simulink model "V2G_Simulator"  (R2021b)
settings: Solver=VariableStepAuto  StartTime=0.0  StopTime=10.0  RelTol=1e-3
settings Model: Creator=The MathWorks, Inc.  LastModifiedBy=rhdej

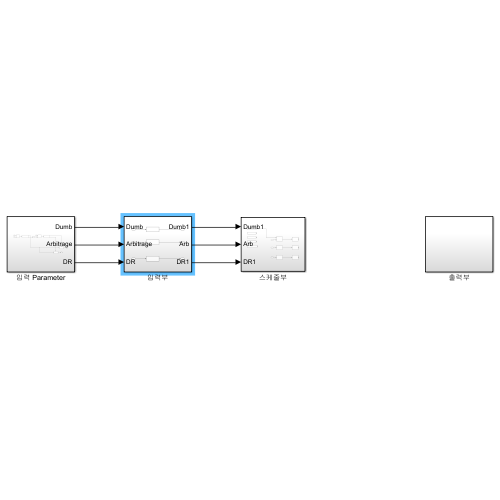
[thumbnail: Simulink's stored preview of the top-level diagram]
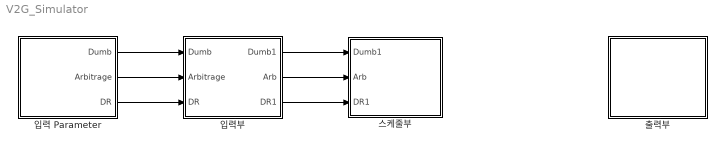
== system V2G_Simulator ==
  스케줄부 : Subsystem
  입력 Parameter : Subsystem
  입력부 : Subsystem
  출력부 : Subsystem
  wires:
  입력부/1(Dumb1) -> 스케줄부/1(Dumb1)
  입력부/2(Arb) -> 스케줄부/2(Arb)
  입력부/3(DR1) -> 스케줄부/3(DR1)
  입력 Parameter/1(Dumb) -> 입력부/1(Dumb)
  입력 Parameter/2(Arbitrage) -> 입력부/2(Arbitrage)
  입력 Parameter/3(DR) -> 입력부/3(DR)

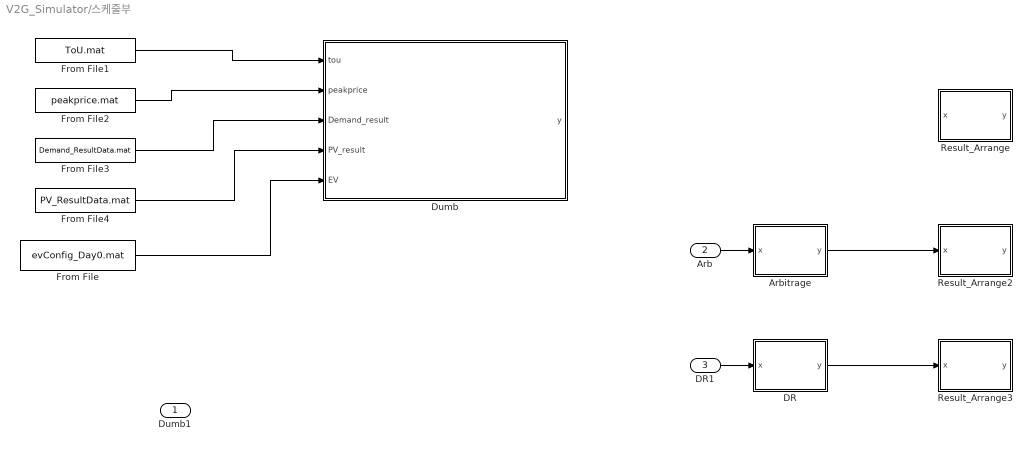
== system V2G_Simulator/스케줄부 ==
  Dumb1 : Inport
  Arb : Inport  Port=2
  DR1 : Inport  Port=3
  Arbitrage : MATLAB Function  TreatAsAtomicUnit=on
  DR : MATLAB Function  TreatAsAtomicUnit=on
  Dumb : MATLAB Function  TreatAsAtomicUnit=on
  From File : FromFile  FileName=evConfig_Day0.mat  SampleTime=0
  From File1 : FromFile  FileName=ToU.mat  SampleTime=0
  From File2 : FromFile  FileName=peakprice.mat  SampleTime=0
  From File3 : FromFile  FileName=Demand_ResultData.mat  SampleTime=0
  From File4 : FromFile  FileName=PV_ResultData.mat  SampleTime=0
  Result_Arrange : MATLAB Function  TreatAsAtomicUnit=on
  Result_Arrange2 : MATLAB Function  TreatAsAtomicUnit=on
  Result_Arrange3 : MATLAB Function  TreatAsAtomicUnit=on
  wires:
  Arbitrage/1(y) -> Result_Arrange2/1(x)
  DR/1(y) -> Result_Arrange3/1(x)
  Arb/1 -> Arbitrage/1(x)
  DR1/1 -> DR/1(x)
  From File1/1 -> Dumb/1(tou)
  From File2/1 -> Dumb/2(peakprice)
  From File3/1 -> Dumb/3(Demand_result)
  From File4/1 -> Dumb/4(PV_result)
  From File/1 -> Dumb/5(EV)

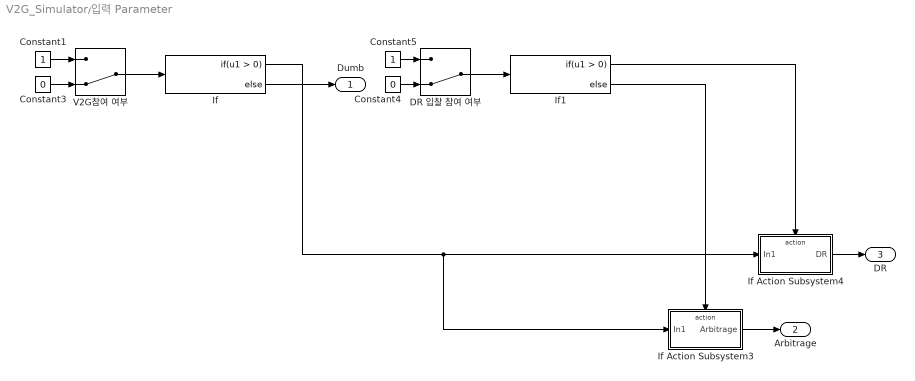
== system V2G_Simulator/입력 Parameter ==
  Constant1 : Constant
  Constant3 : Constant  Value=0
  Constant4 : Constant  Value=0
  Constant5 : Constant
  DR 입찰 참여 여부 : ManualSwitch  CurrentSetting=0
  If : If
  If Action Subsystem3 : Subsystem  TreatAsAtomicUnit=on
  If Action Subsystem4 : Subsystem  TreatAsAtomicUnit=on
  If1 : If
  V2G참여 여부 : ManualSwitch  CurrentSetting=0
  Dumb : Outport
  Arbitrage : Outport  Port=2
  DR : Outport  Port=3
  wires:
  Constant3/1 -> V2G참여 여부/2
  Constant1/1 -> V2G참여 여부/1
  V2G참여 여부/1 -> If/1
  If/2 -> Dumb/1
  Constant4/1 -> DR 입찰 참여 여부/2
  Constant5/1 -> DR 입찰 참여 여부/1
  DR 입찰 참여 여부/1 -> If1/1
  If/1 -> If Action Subsystem4/1(In1), If Action Subsystem3/1(In1)
  If1/2 -> If Action Subsystem3/Action
  If Action Subsystem4/1(DR) -> DR/1
  If Action Subsystem3/1(Arbitrage) -> Arbitrage/1
  If1/1 -> If Action Subsystem4/Action

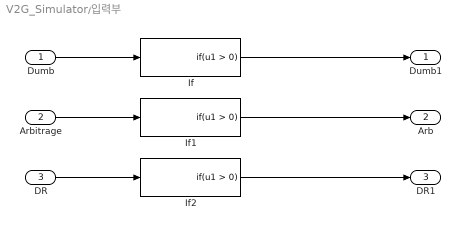
== system V2G_Simulator/입력부 ==
  Dumb : Inport
  Arbitrage : Inport  Port=2
  DR : Inport  Port=3
  If : If  ShowElse=off
  If1 : If  ShowElse=off
  If2 : If  ShowElse=off
  Dumb1 : Outport
  Arb : Outport  Port=2
  DR1 : Outport  Port=3
  wires:
  Dumb/1 -> If/1
  Arbitrage/1 -> If1/1
  DR/1 -> If2/1
  If/1 -> Dumb1/1
  If1/1 -> Arb/1
  If2/1 -> DR1/1

== system V2G_Simulator/출력부 ==

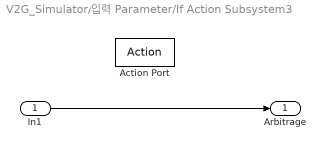
== system V2G_Simulator/입력 Parameter/If Action Subsystem3 ==
  In1 : Inport
  Action Port : ActionPort  ActionPortLabel=else
  Arbitrage : Outport
  wires:
  In1/1 -> Arbitrage/1

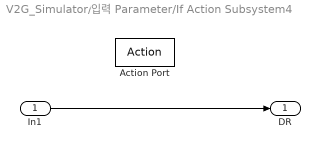
== system V2G_Simulator/입력 Parameter/If Action Subsystem4 ==
  In1 : Inport
  Action Port : ActionPort  ActionPortLabel=if(u1 > 0)
  DR : Outport
  wires:
  In1/1 -> DR/1

== matlab function V2G_Simulator/스케줄부/Arbitrage ==
  data: x input; y output
function y = temp(x)


end

== matlab function V2G_Simulator/스케줄부/DR ==
  data: x input; y output
function y = temp(x)

== matlab function V2G_Simulator/스케줄부/Dumb ==
  data: tou input; y output; peakprice input; Demand_result input; PV_result input; EV input
function y = temp(tou, peakprice, Demand_result, PV_result, EV)

coder.extrinsic("intlinprog")

x = [0]


end

== matlab function V2G_Simulator/스케줄부/Result_Arrange ==
  data: x input; y output
function y = temp(x)

== matlab function V2G_Simulator/스케줄부/Result_Arrange2 ==
  data: x input; y output
function y = temp(x)

== matlab function V2G_Simulator/스케줄부/Result_Arrange3 ==
  data: x input; y output
function y = temp(x)
